simulink library "CTRL_TRGT"  (R2023b)
settings: Solver=VariableStepAuto  StartTime=0.0  StopTime=10.0  RelTol=1e-3
libraries: CTRL_TRGT_DEC x1, CTRL_TRGT_SADES x1, CTRL_TRGT_SAUPPB x1, CTRL_TRGT_UG x1, CTRL_TRGT_YRDES x1, CTRL_TRGT_YRUPPB x1
settings Model: Creator=blatak  LastModifiedBy=blatak

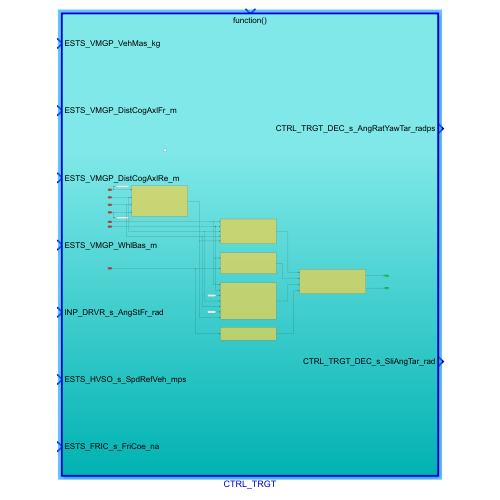
[thumbnail: Simulink's stored preview of the top-level diagram]
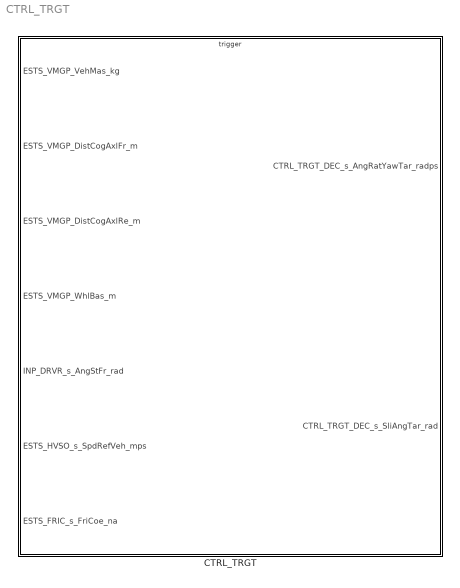
== system CTRL_TRGT ==
  CTRL_TRGT : Subsystem  TreatAsAtomicUnit=on

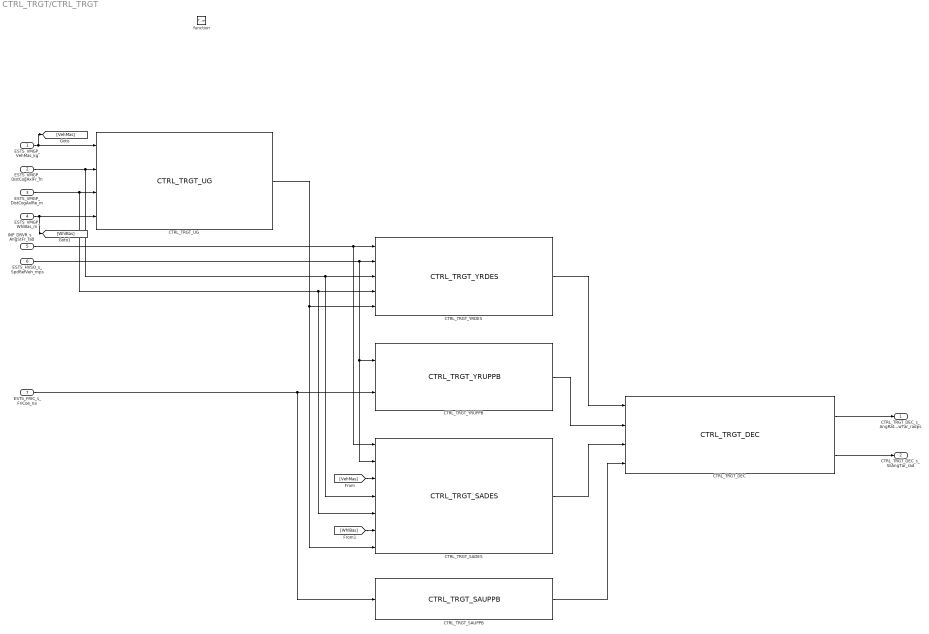
== system CTRL_TRGT/CTRL_TRGT ==
  ESTS_VMGP_VehMas_kg : Inport
  ESTS_VMGP_DistCogAxlFr_m : Inport  Port=2
  ESTS_VMGP_DistCogAxlRe_m : Inport  Port=3
  ESTS_VMGP_WhlBas_m : Inport  Port=4
  INP_DRVR_s_AngStFr_rad : Inport  Port=5
  ESTS_HVSO_s_SpdRefVeh_mps : Inport  Port=6
  ESTS_FRIC_s_FriCoe_na : Inport  Port=7
  function : TriggerPort  TriggerType=function-call  VariantControl=(inherit)
  CTRL_TRGT_DEC : CTRL_TRGT_DEC/CTRL_TRGT_DEC  SystemSampleTime=-1  VariantActivationTime=update diagram  AllowFlexibleInterface=on  Latency=0  AutoFrameSizeCalculation=off
  CTRL_TRGT_SADES : CTRL_TRGT_SADES/CTRL_TRGT_SADES  SystemSampleTime=-1  VariantActivationTime=update diagram  AllowFlexibleInterface=on  Latency=0  AutoFrameSizeCalculation=off
  CTRL_TRGT_SAUPPB : CTRL_TRGT_SAUPPB/CTRL_TRGT_SAUPPB  SystemSampleTime=-1  VariantActivationTime=update diagram  AllowFlexibleInterface=on  Latency=0  AutoFrameSizeCalculation=off
  CTRL_TRGT_UG : CTRL_TRGT_UG/CTRL_TRGT_UG  SystemSampleTime=-1  VariantActivationTime=update diagram  AllowFlexibleInterface=on  Latency=0  AutoFrameSizeCalculation=off
  CTRL_TRGT_YRDES : CTRL_TRGT_YRDES/CTRL_TRGT_YRDES  SystemSampleTime=-1  VariantActivationTime=update diagram  AllowFlexibleInterface=on  Latency=0  AutoFrameSizeCalculation=off
  CTRL_TRGT_YRUPPB : CTRL_TRGT_YRUPPB/CTRL_TRGT_YRUPPB  SystemSampleTime=-1  VariantActivationTime=update diagram  AllowFlexibleInterface=on  Latency=0  AutoFrameSizeCalculation=off
  CTRL_TRGT_DEC_s_AngRatYawTar_radps : Outport
  CTRL_TRGT_DEC_s_SliAngTar_rad : Outport  Port=2
  wires:
  ESTS_VMGP_VehMas_kg/1 -> [VehMas], CTRL_TRGT_UG/1
  ESTS_VMGP_WhlBas_m/1 -> [WhlBas], CTRL_TRGT_UG/4
  ESTS_HVSO_s_SpdRefVeh_mps/1 -> CTRL_TRGT_YRUPPB/1, CTRL_TRGT_SADES/2, CTRL_TRGT_YRDES/2
  CTRL_TRGT_UG/1 -> CTRL_TRGT_YRDES/5, CTRL_TRGT_SADES/7
  INP_DRVR_s_AngStFr_rad/1 -> CTRL_TRGT_SADES/1, CTRL_TRGT_YRDES/1
  ESTS_FRIC_s_FriCoe_na/1 -> CTRL_TRGT_YRUPPB/2, CTRL_TRGT_SAUPPB/1
  ESTS_VMGP_DistCogAxlFr_m/1 -> CTRL_TRGT_UG/2, CTRL_TRGT_YRDES/3, CTRL_TRGT_SADES/4
  ESTS_VMGP_DistCogAxlRe_m/1 -> CTRL_TRGT_YRDES/4, CTRL_TRGT_SADES/5, CTRL_TRGT_UG/3
  [VehMas] -> CTRL_TRGT_SADES/3
  [WhlBas] -> CTRL_TRGT_SADES/6
  CTRL_TRGT_YRDES/1 -> CTRL_TRGT_DEC/1
  CTRL_TRGT_YRUPPB/1 -> CTRL_TRGT_DEC/2
  CTRL_TRGT_SADES/1 -> CTRL_TRGT_DEC/3
  CTRL_TRGT_SAUPPB/1 -> CTRL_TRGT_DEC/4
  CTRL_TRGT_DEC/1 -> CTRL_TRGT_DEC_s_AngRatYawTar_radps/1
  CTRL_TRGT_DEC/2 -> CTRL_TRGT_DEC_s_SliAngTar_rad/1
